simulink model "Image_to_output"  (R2023b)
settings: Solver=VariableStepAuto  StartTime=0.0  StopTime=10.0  RelTol=1e-3
libraries: visionsources x20, deeplib x1, audiofeatures x1
settings Model: Creator=TKM  LastModifiedBy=shitosu

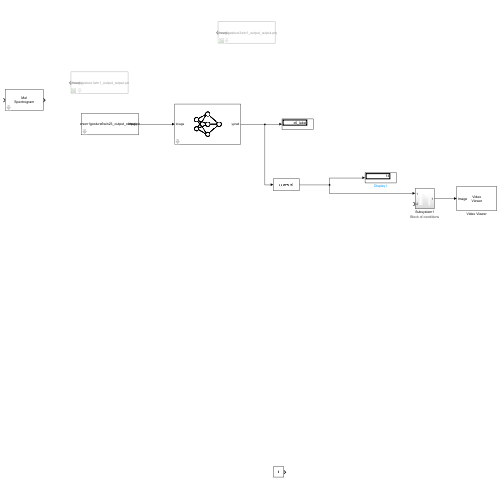
[thumbnail: Simulink's stored preview of the top-level diagram]
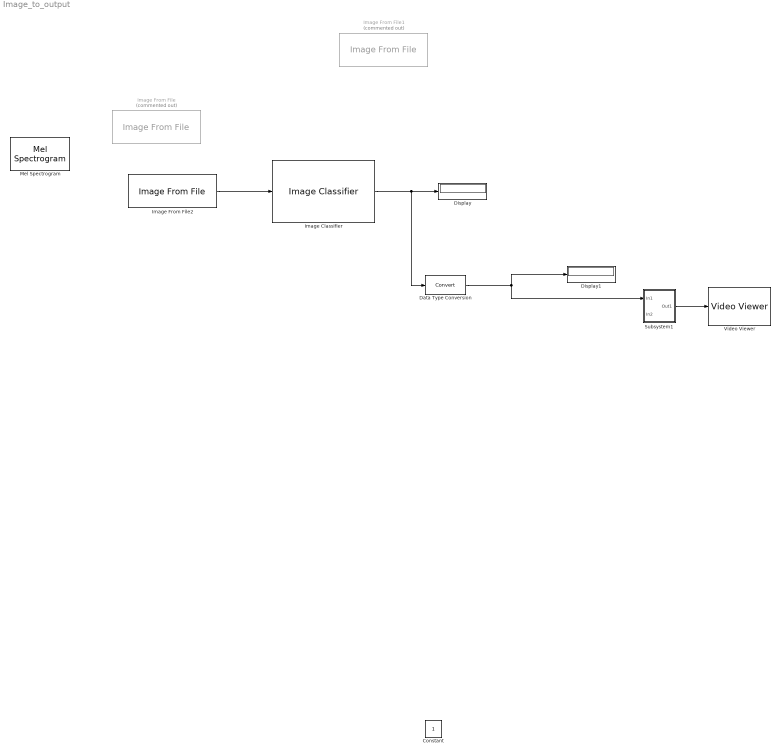
== system Image_to_output ==
  Constant : Constant
  Data Type Conversion : DataTypeConversion  RndMeth=Simplest  SaturateOnIntegerOverflow=off
  Display : Display
  Display1 : Display
  Image Classifier : deeplib/Image Classifier  Network=Network from MAT-file  NetworkFunction=squeezenet  NetworkFilePath=C:\Users\shitosu\Downloads\Trained Network Resnet50 full.mat  MiniBatchSize=128  ResizeInput=on  Classification=on  Predictions=off  ForceInterpretedSim=off  PredictMode=All probabilities and labels  K=5
  Image From File : visionsources/Image From File  Tag=vipblks_nd  Commented=on  FileName=D:\Gest224\1\person1gesture1win1_output_output.png  Ts=inf  imagePorts=One multidimensional signal  OutPortLabels=R|G|B  ImageDataType=Inherit from input image  sdImageDataType=uint(8)  Signed=on  WordLength=16  FractionLengthMode=User-defined  FractionLength=15
  Image From File1 : visionsources/Image From File  Tag=vipblks_nd  Commented=on  FileName=D:\Gest224\2\person1gesture2win1_output_output.png  Ts=inf  imagePorts=One multidimensional signal  OutPortLabels=R|G|B  ImageDataType=Inherit from input image  sdImageDataType=uint(8)  Signed=on  WordLength=16  FractionLengthMode=User-defined  FractionLength=15
  Image From File2 : visionsources/Image From File  Tag=vipblks_nd  FileName=C:\Users\shitosu\Desktop\Mini_dataset\6_r\person1gesture6win23_output_output.png  Ts=inf  imagePorts=One multidimensional signal  OutPortLabels=R|G|B  ImageDataType=Inherit from input image  sdImageDataType=uint(8)  Signed=on  WordLength=16  FractionLengthMode=User-defined  FractionLength=15
  Mel Spectrogram : audiofeatures/Mel Spectrogram  FrequencyScale=mel  AutoNumBands=off  NumBands=32  AutoFrequencyRange=on  FrequencyRange=[0, 22050]  FilterBankDesignDomain=linear  FilterBankNormalization=bandwidth  MelStyle=oshaughnessy  OutputFrequencyVector=off  WindowParameter=hamming(1024,'periodic')  WindowNormalization=on  OverlapLength=512  AutoFFTLength=on  FFTLength=1024  SpectrumType=magnitude  NumHops=1  NumHopsOverlap=0  InheritSampleRate=off  SampleRate=44.1e3
  Subsystem1 : Subsystem
      settings: AttributesFormatString=Block of conditions
  Video Viewer : VideoViewer  FigPos=[330.6 692.4 418.4 304]
  wires:
  Data Type Conversion/1 -> Display1/1, Subsystem1/1(In1)
  Image From File2/1 -> Image Classifier/1
  Subsystem1/1(Out1) -> Video Viewer/1
  Image Classifier/1 -> Data Type Conversion/1, Display/1

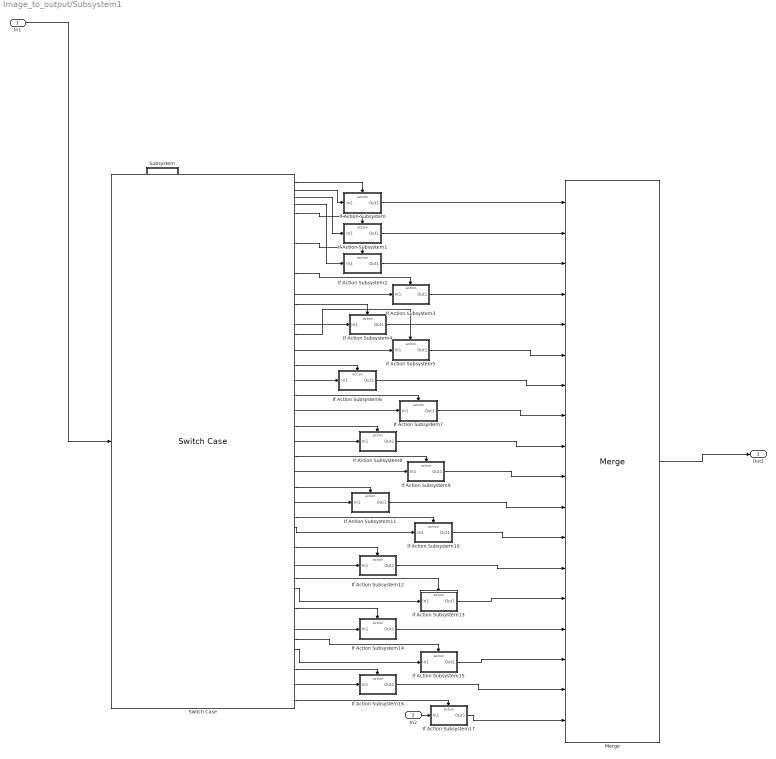
== system Image_to_output/Subsystem1 ==
  In1 : Inport
  In2 : Inport  Port=2
  If Action Subsystem : Subsystem  TreatAsAtomicUnit=on
  If Action Subsystem1 : Subsystem  TreatAsAtomicUnit=on
  If Action Subsystem10 : Subsystem  TreatAsAtomicUnit=on
  If Action Subsystem11 : Subsystem  TreatAsAtomicUnit=on
  If Action Subsystem12 : Subsystem  TreatAsAtomicUnit=on
  If Action Subsystem13 : Subsystem  TreatAsAtomicUnit=on
  If Action Subsystem14 : Subsystem  TreatAsAtomicUnit=on
  If Action Subsystem15 : Subsystem  TreatAsAtomicUnit=on
  If Action Subsystem16 : Subsystem  TreatAsAtomicUnit=on
  If Action Subsystem17 : Subsystem  TreatAsAtomicUnit=on
  If Action Subsystem2 : Subsystem  TreatAsAtomicUnit=on
  If Action Subsystem3 : Subsystem  TreatAsAtomicUnit=on
  If Action Subsystem4 : Subsystem  TreatAsAtomicUnit=on
  If Action Subsystem5 : Subsystem  TreatAsAtomicUnit=on
  If Action Subsystem6 : Subsystem  TreatAsAtomicUnit=on
  If Action Subsystem7 : Subsystem  TreatAsAtomicUnit=on
  If Action Subsystem8 : Subsystem  TreatAsAtomicUnit=on
  If Action Subsystem9 : Subsystem  TreatAsAtomicUnit=on
  Merge : Merge  Inputs=18  InitialOutput=1
  Subsystem : Subsystem
  Switch Case : SwitchCase  CaseConditions={1,10,11,12,13,14,15,16,17,2,3,4,5,6,7,8,9}
  Out1 : Outport
  wires:
  Switch Case/11 -> If Action Subsystem11/Action
  If Action Subsystem4/1(Out1) -> Merge/5
  Subsystem/11(Out11) -> If Action Subsystem11/1(In1)
  Merge/1 -> Out1/1
  If Action Subsystem11/1(Out1) -> Merge/11
  Subsystem/10(Out10) -> If Action Subsystem9/1(In1)
  If Action Subsystem3/1(Out1) -> Merge/4
  Switch Case/13 -> If Action Subsystem12/Action
  If Action Subsystem8/1(Out1) -> Merge/9
  Subsystem/13(Out13) -> If Action Subsystem12/1(In1)
  If Action Subsystem5/1(Out1) -> Merge/6
  Switch Case/7 -> If Action Subsystem6/Action
  Switch Case/8 -> If Action Subsystem7/Action
  Subsystem/14(Out14) -> If Action Subsystem13/1(In1)
  If Action Subsystem7/1(Out1) -> Merge/8
  Switch Case/6 -> If Action Subsystem5/Action
  If Action Subsystem10/1(Out1) -> Merge/12
  Subsystem/17(Out17) -> If Action Subsystem16/1(In1)
  Switch Case/3 -> If Action Subsystem2/Action
  Switch Case/5 -> If Action Subsystem4/Action
  If Action Subsystem16/1(Out1) -> Merge/17
  Switch Case/2 -> If Action Subsystem1/Action
  Subsystem/2(Out2) -> If Action Subsystem1/1(In1)
  Switch Case/1 -> If Action Subsystem/Action
  Switch Case/18 -> If Action Subsystem17/Action
  If Action Subsystem13/1(Out1) -> Merge/14
  Switch Case/12 -> If Action Subsystem10/Action
  If Action Subsystem2/1(Out1) -> Merge/3
  If Action Subsystem15/1(Out1) -> Merge/16
  If Action Subsystem14/1(Out1) -> Merge/15
  Subsystem/4(Out4) -> If Action Subsystem3/1(In1)
  Subsystem/6(Out6) -> If Action Subsystem5/1(In1)
  Subsystem/9(Out9) -> If Action Subsystem8/1(In1)
  In2/1 -> If Action Subsystem17/1(In1)
  If Action Subsystem6/1(Out1) -> Merge/7
  Switch Case/10 -> If Action Subsystem9/Action
  Subsystem/12(Out12) -> If Action Subsystem10/1(In1)
  Switch Case/9 -> If Action Subsystem8/Action
  Switch Case/16 -> If Action Subsystem15/Action
  Subsystem/15(Out15) -> If Action Subsystem14/1(In1)
  If Action Subsystem12/1(Out1) -> Merge/13
  Subsystem/8(Out8) -> If Action Subsystem7/1(In1)
  If Action Subsystem9/1(Out1) -> Merge/10
  Switch Case/15 -> If Action Subsystem14/Action
  Switch Case/17 -> If Action Subsystem16/Action
  If Action Subsystem17/1(Out1) -> Merge/18
  Subsystem/16(Out16) -> If Action Subsystem15/1(In1)
  Subsystem/5(Out5) -> If Action Subsystem4/1(In1)
  If Action Subsystem1/1(Out1) -> Merge/2
  Switch Case/4 -> If Action Subsystem3/Action
  If Action Subsystem/1(Out1) -> Merge/1
  Subsystem/1(Out1) -> If Action Subsystem/1(In1)
  Subsystem/7(Out7) -> If Action Subsystem6/1(In1)
  Switch Case/14 -> If Action Subsystem13/Action
  Subsystem/3(Out3) -> If Action Subsystem2/1(In1)
  In1/1 -> Switch Case/1

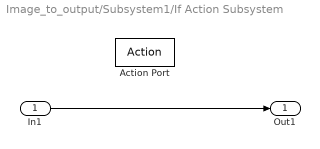
== system Image_to_output/Subsystem1/If Action Subsystem ==
  In1 : Inport
  Action Port : ActionPort  ActionPortLabel=case [ 1 ]:
  Out1 : Outport
  wires:
  In1/1 -> Out1/1

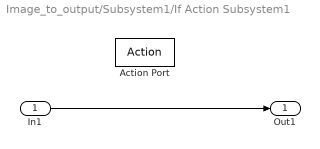
== system Image_to_output/Subsystem1/If Action Subsystem1 ==
  In1 : Inport
  Action Port : ActionPort  ActionPortLabel=case [ 10 ]:
  Out1 : Outport
  wires:
  In1/1 -> Out1/1

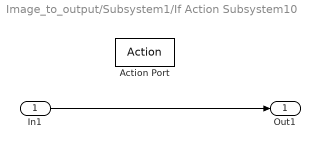
== system Image_to_output/Subsystem1/If Action Subsystem10 ==
  In1 : Inport
  Action Port : ActionPort  ActionPortLabel=case [ 4 ]:
  Out1 : Outport
  wires:
  In1/1 -> Out1/1

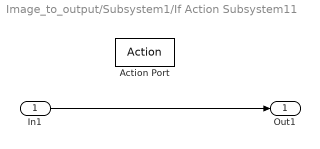
== system Image_to_output/Subsystem1/If Action Subsystem11 ==
  In1 : Inport
  Action Port : ActionPort  ActionPortLabel=case [ 3 ]:
  Out1 : Outport
  wires:
  In1/1 -> Out1/1

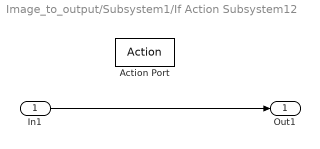
== system Image_to_output/Subsystem1/If Action Subsystem12 ==
  In1 : Inport
  Action Port : ActionPort  ActionPortLabel=case [ 5 ]:
  Out1 : Outport
  wires:
  In1/1 -> Out1/1

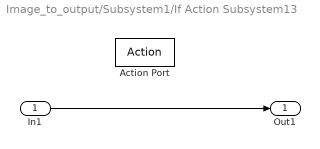
== system Image_to_output/Subsystem1/If Action Subsystem13 ==
  In1 : Inport
  Action Port : ActionPort  ActionPortLabel=case [ 6 ]:
  Out1 : Outport
  wires:
  In1/1 -> Out1/1

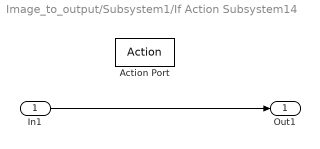
== system Image_to_output/Subsystem1/If Action Subsystem14 ==
  In1 : Inport
  Action Port : ActionPort  ActionPortLabel=case [ 7 ]:
  Out1 : Outport
  wires:
  In1/1 -> Out1/1

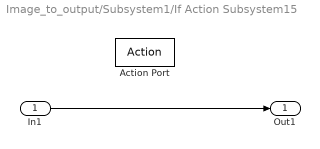
== system Image_to_output/Subsystem1/If Action Subsystem15 ==
  In1 : Inport
  Action Port : ActionPort  ActionPortLabel=case [ 8 ]:
  Out1 : Outport
  wires:
  In1/1 -> Out1/1

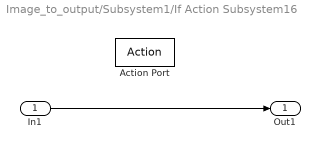
== system Image_to_output/Subsystem1/If Action Subsystem16 ==
  In1 : Inport
  Action Port : ActionPort  ActionPortLabel=case [ 9 ]:
  Out1 : Outport
  wires:
  In1/1 -> Out1/1

== system Image_to_output/Subsystem1/If Action Subsystem17 ==
  In1 : Inport
  Action Port : ActionPort  ActionPortLabel=default:
  Out1 : Outport
  wires:
  In1/1 -> Out1/1

== system Image_to_output/Subsystem1/If Action Subsystem2 ==
  In1 : Inport
  Action Port : ActionPort  ActionPortLabel=case [ 11 ]:
  Out1 : Outport
  wires:
  In1/1 -> Out1/1

== system Image_to_output/Subsystem1/If Action Subsystem3 ==
  In1 : Inport
  Action Port : ActionPort  ActionPortLabel=case [ 12 ]:
  Out1 : Outport
  wires:
  In1/1 -> Out1/1

== system Image_to_output/Subsystem1/If Action Subsystem4 ==
  In1 : Inport
  Action Port : ActionPort  ActionPortLabel=case [ 13 ]:
  Out1 : Outport
  wires:
  In1/1 -> Out1/1

== system Image_to_output/Subsystem1/If Action Subsystem5 ==
  In1 : Inport
  Action Port : ActionPort  ActionPortLabel=case [ 14 ]:
  Out1 : Outport
  wires:
  In1/1 -> Out1/1

== system Image_to_output/Subsystem1/If Action Subsystem6 ==
  In1 : Inport
  Action Port : ActionPort  ActionPortLabel=case [ 15 ]:
  Out1 : Outport
  wires:
  In1/1 -> Out1/1

== system Image_to_output/Subsystem1/If Action Subsystem7 ==
  In1 : Inport
  Action Port : ActionPort  ActionPortLabel=case [ 16 ]:
  Out1 : Outport
  wires:
  In1/1 -> Out1/1

== system Image_to_output/Subsystem1/If Action Subsystem8 ==
  In1 : Inport
  Action Port : ActionPort  ActionPortLabel=case [ 17 ]:
  Out1 : Outport
  wires:
  In1/1 -> Out1/1

== system Image_to_output/Subsystem1/If Action Subsystem9 ==
  In1 : Inport
  Action Port : ActionPort  ActionPortLabel=case [ 2 ]:
  Out1 : Outport
  wires:
  In1/1 -> Out1/1

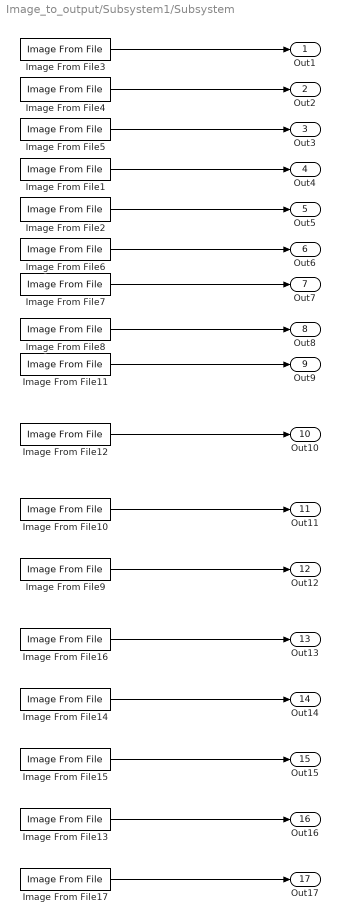
== system Image_to_output/Subsystem1/Subsystem ==
  Image From File1 : visionsources/Image From File  Tag=vipblks_nd  FileName=C:\Users\shitosu\Desktop\Matlab\image_part_004.jpg  Ts=inf  imagePorts=One multidimensional signal  OutPortLabels=R|G|B  ImageDataType=Inherit from input image  sdImageDataType=uint(8)  Signed=on  WordLength=16  FractionLengthMode=User-defined  FractionLength=15
  Image From File10 : visionsources/Image From File  Tag=vipblks_nd  FileName=C:\Users\shitosu\Desktop\Matlab\image_part_011.jpg  Ts=inf  imagePorts=One multidimensional signal  OutPortLabels=R|G|B  ImageDataType=Inherit from input image  sdImageDataType=uint(8)  Signed=on  WordLength=16  FractionLengthMode=User-defined  FractionLength=15
  Image From File11 : visionsources/Image From File  Tag=vipblks_nd  FileName=C:\Users\shitosu\Desktop\Matlab\image_part_009.jpg  Ts=inf  imagePorts=One multidimensional signal  OutPortLabels=R|G|B  ImageDataType=Inherit from input image  sdImageDataType=uint(8)  Signed=on  WordLength=16  FractionLengthMode=User-defined  FractionLength=15
  Image From File12 : visionsources/Image From File  Tag=vipblks_nd  FileName=C:\Users\shitosu\Desktop\Matlab\image_part_010.jpg  Ts=inf  imagePorts=One multidimensional signal  OutPortLabels=R|G|B  ImageDataType=Inherit from input image  sdImageDataType=uint(8)  Signed=on  WordLength=16  FractionLengthMode=User-defined  FractionLength=15
  Image From File13 : visionsources/Image From File  Tag=vipblks_nd  FileName=C:\Users\shitosu\Desktop\Matlab\image_part_016.jpg  Ts=inf  imagePorts=One multidimensional signal  OutPortLabels=R|G|B  ImageDataType=Inherit from input image  sdImageDataType=uint(8)  Signed=on  WordLength=16  FractionLengthMode=User-defined  FractionLength=15
  Image From File14 : visionsources/Image From File  Tag=vipblks_nd  FileName=C:\Users\shitosu\Desktop\Matlab\image_part_014.jpg  Ts=inf  imagePorts=One multidimensional signal  OutPortLabels=R|G|B  ImageDataType=Inherit from input image  sdImageDataType=uint(8)  Signed=on  WordLength=16  FractionLengthMode=User-defined  FractionLength=15
  Image From File15 : visionsources/Image From File  Tag=vipblks_nd  FileName=C:\Users\shitosu\Desktop\Matlab\image_part_015.jpg  Ts=inf  imagePorts=One multidimensional signal  OutPortLabels=R|G|B  ImageDataType=Inherit from input image  sdImageDataType=uint(8)  Signed=on  WordLength=16  FractionLengthMode=User-defined  FractionLength=15
  Image From File16 : visionsources/Image From File  Tag=vipblks_nd  FileName=C:\Users\shitosu\Desktop\Matlab\image_part_013.jpg  Ts=inf  imagePorts=One multidimensional signal  OutPortLabels=R|G|B  ImageDataType=Inherit from input image  sdImageDataType=uint(8)  Signed=on  WordLength=16  FractionLengthMode=User-defined  FractionLength=15
  Image From File17 : visionsources/Image From File  Tag=vipblks_nd  FileName=C:\Users\shitosu\Desktop\Matlab\image_part_012.jpg  Ts=inf  imagePorts=One multidimensional signal  OutPortLabels=R|G|B  ImageDataType=Inherit from input image  sdImageDataType=uint(8)  Signed=on  WordLength=16  FractionLengthMode=User-defined  FractionLength=15
  Image From File2 : visionsources/Image From File  Tag=vipblks_nd  FileName=C:\Users\shitosu\Desktop\Matlab\image_part_005.jpg  Ts=inf  imagePorts=One multidimensional signal  OutPortLabels=R|G|B  ImageDataType=Inherit from input image  sdImageDataType=uint(8)  Signed=on  WordLength=16  FractionLengthMode=User-defined  FractionLength=15
  Image From File3 : visionsources/Image From File  Tag=vipblks_nd  FileName=C:\Users\shitosu\Desktop\Matlab\image_part_001.jpg  Ts=inf  imagePorts=One multidimensional signal  OutPortLabels=R|G|B  ImageDataType=Inherit from input image  sdImageDataType=uint(8)  Signed=on  WordLength=16  FractionLengthMode=User-defined  FractionLength=15
  Image From File4 : visionsources/Image From File  Tag=vipblks_nd  FileName=C:\Users\shitosu\Desktop\Matlab\image_part_002.jpg  Ts=inf  imagePorts=One multidimensional signal  OutPortLabels=R|G|B  ImageDataType=Inherit from input image  sdImageDataType=uint(8)  Signed=on  WordLength=16  FractionLengthMode=User-defined  FractionLength=15
  Image From File5 : visionsources/Image From File  Tag=vipblks_nd  FileName=C:\Users\shitosu\Desktop\Matlab\image_part_003.jpg  Ts=inf  imagePorts=One multidimensional signal  OutPortLabels=R|G|B  ImageDataType=Inherit from input image  sdImageDataType=uint(8)  Signed=on  WordLength=16  FractionLengthMode=User-defined  FractionLength=15
  Image From File6 : visionsources/Image From File  Tag=vipblks_nd  FileName=C:\Users\shitosu\Desktop\Matlab\image_part_006.jpg  Ts=inf  imagePorts=One multidimensional signal  OutPortLabels=R|G|B  ImageDataType=Inherit from input image  sdImageDataType=uint(8)  Signed=on  WordLength=16  FractionLengthMode=User-defined  FractionLength=15
  Image From File7 : visionsources/Image From File  Tag=vipblks_nd  FileName=C:\Users\shitosu\Desktop\Matlab\image_part_007.jpg  Ts=inf  imagePorts=One multidimensional signal  OutPortLabels=R|G|B  ImageDataType=Inherit from input image  sdImageDataType=uint(8)  Signed=on  WordLength=16  FractionLengthMode=User-defined  FractionLength=15
  Image From File8 : visionsources/Image From File  Tag=vipblks_nd  FileName=C:\Users\shitosu\Desktop\Matlab\image_part_008.jpg  Ts=inf  imagePorts=One multidimensional signal  OutPortLabels=R|G|B  ImageDataType=Inherit from input image  sdImageDataType=uint(8)  Signed=on  WordLength=16  FractionLengthMode=User-defined  FractionLength=15
  Image From File9 : visionsources/Image From File  Tag=vipblks_nd  FileName=C:\Users\shitosu\Desktop\Matlab\image_part_012.jpg  Ts=inf  imagePorts=One multidimensional signal  OutPortLabels=R|G|B  ImageDataType=Inherit from input image  sdImageDataType=uint(8)  Signed=on  WordLength=16  FractionLengthMode=User-defined  FractionLength=15
  Out1 : Outport
  Out2 : Outport  Port=2
  Out3 : Outport  Port=3
  Out4 : Outport  Port=4
  Out5 : Outport  Port=5
  Out6 : Outport  Port=6
  Out7 : Outport  Port=7
  Out8 : Outport  Port=8
  Out9 : Outport  Port=9
  Out10 : Outport  Port=10
  Out11 : Outport  Port=11
  Out12 : Outport  Port=12
  Out13 : Outport  Port=13
  Out14 : Outport  Port=14
  Out15 : Outport  Port=15
  Out16 : Outport  Port=16
  Out17 : Outport  Port=17
  wires:
  Image From File4/1 -> Out2/1
  Image From File3/1 -> Out1/1
  Image From File5/1 -> Out3/1
  Image From File1/1 -> Out4/1
  Image From File6/1 -> Out6/1
  Image From File2/1 -> Out5/1
  Image From File10/1 -> Out11/1
  Image From File12/1 -> Out10/1
  Image From File9/1 -> Out12/1
  Image From File7/1 -> Out7/1
  Image From File11/1 -> Out9/1
  Image From File8/1 -> Out8/1
  Image From File15/1 -> Out15/1
  Image From File17/1 -> Out17/1
  Image From File13/1 -> Out16/1
  Image From File14/1 -> Out14/1
  Image From File16/1 -> Out13/1
